simulink model "CE141IntroModel2"  (R2014b)
settings: Solver=ode45  StartTime=0.0  StopTime=40  MaxStep=0.1  RelTol=1e-3
settings Model: Creator=Dejan  LastModifiedBy=Dejan
settings DataIOCC: SignalLoggingSaveFormat=ModelDataLogs
settings OptimizationCC: ExpressionDepthLimit=2147483647
settings DebuggingCC: UnderspecifiedInitializationDetection=Classic  MergeDetectMultiDrivingBlocksExec=none  SolverPrmCheckMsg=none  FcnCallInpInsideContextMsg=EnableAllAsWarning  StateNameClashWarn=warning
settings GRTTargetCC: CombineOutputUpdateFcns=off  GRTInterface=on

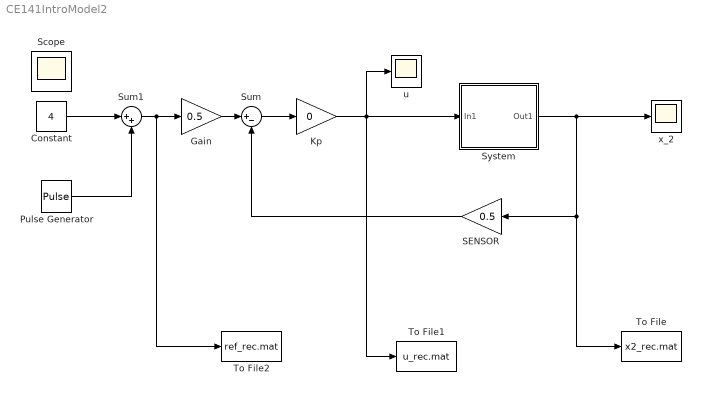
== system CE141IntroModel2 ==
  Constant : Constant  Value=4
  Gain : Gain  Gain=0.5
  Kp : Gain  Gain=0
  Pulse Generator : DiscretePulseGenerator  PulseType=Time based  Amplitude=1.4  Period=10  PulseWidth=50  PhaseDelay=5
  SENSOR : Gain  Gain=0.5
  Sum : Sum  Inputs=|+-
  Sum1 : Sum  Inputs=|++
  System : Subsystem
  To File : ToFile  Filename=x2_rec.mat  MatrixName=x2_rec  SaveFormat=Timeseries
  To File1 : ToFile  Filename=u_rec.mat  MatrixName=u_rec  SaveFormat=Timeseries
  To File2 : ToFile  Filename=ref_rec.mat  MatrixName=ref_rec  SaveFormat=Timeseries
  u : Scope
  x_2 : Scope
      settings: TimeRange=4  YMin=-3.65625  YMax=0.3437500000000004
  Scope : Scope
      settings: MaxDataPoints=7500
  wires:
  System/1(Out1) -> x_2/1, SENSOR/1, To File/1
  Kp/1 -> System/1(In1), u/1, To File1/1
  SENSOR/1 -> Sum/2
  Gain/1 -> Sum/1
  Sum/1 -> Kp/1
  Pulse Generator/1 -> Sum1/2
  Constant/1 -> Sum1/1
  Sum1/1 -> Gain/1, To File2/1

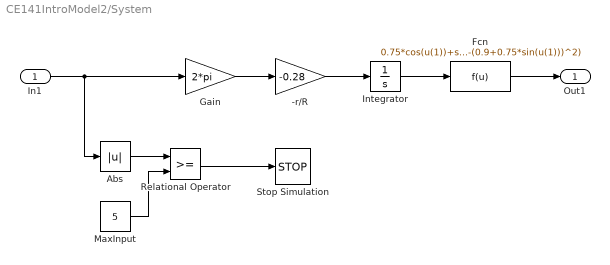
== system CE141IntroModel2/System ==
  In1 : Inport
  -r/R : Gain  Gain=-0.28
  Abs : Abs
  Fcn : Fcn  Expr=0.75*cos(u(1))+sqrt(4.8^2-(0.9+0.75*sin(u(1)))^2)
  Gain : Gain  Gain=2*pi
  Integrator : Integrator  InitialCondition=1
  MaxInput : Constant  Value=5
  Relational Operator : RelationalOperator  OutDataTypeStr=boolean
  Stop Simulation : Stop
  Out1 : Outport
  wires:
  Integrator/1 -> Fcn/1
  Fcn/1 -> Out1/1
  Gain/1 -> -r/R/1
  -r/R/1 -> Integrator/1
  Relational Operator/1 -> Stop Simulation/1
  In1/1 -> Abs/1, Gain/1
  Abs/1 -> Relational Operator/1
  MaxInput/1 -> Relational Operator/2
